simulink library "SEN"  (Simulink 10.2)
settings: Solver=VariableStepAuto  StartTime=0.0  StopTime=10.0  RelTol=1e-3
libraries: SEN_GYR x1, SEN_MTM x1, SEN_SPC x1, SEN_SUN x1
settings Model: Creator=dbell44  LastModifiedBy=dbell44

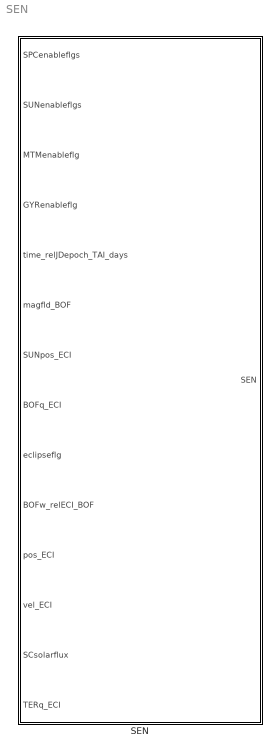
== system SEN ==
  SEN : Subsystem

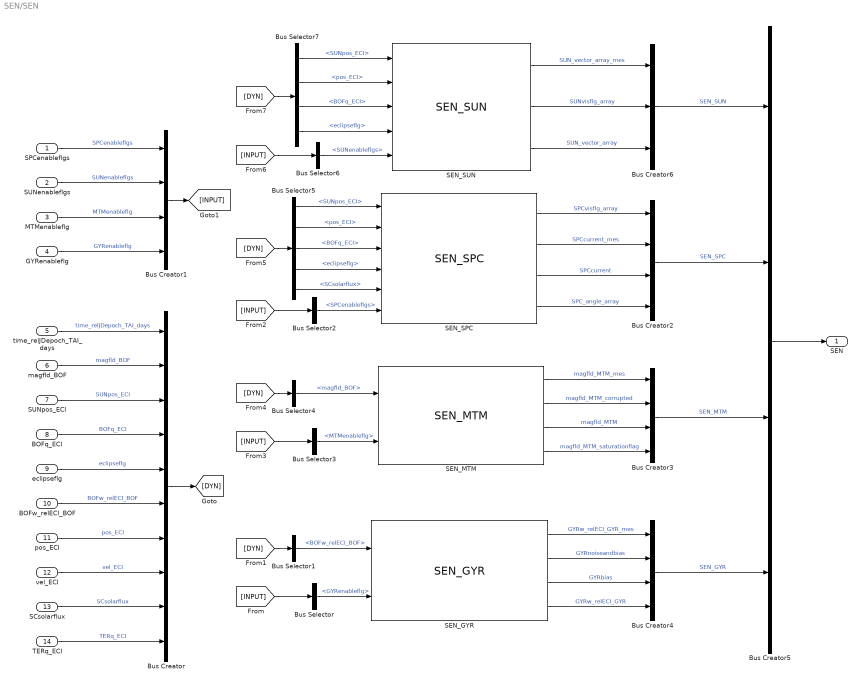
== system SEN/SEN ==
  SPCenableflgs : Inport
  SUNenableflgs : Inport  Port=2
  MTMenableflg : Inport  Port=3
  GYRenableflg : Inport  Port=4
  time_relJDepoch_TAI_days : Inport  Port=5
  magfld_BOF : Inport  Port=6
  SUNpos_ECI : Inport  Port=7
  BOFq_ECI : Inport  Port=8
  eclipseflg : Inport  Port=9
  BOFw_relECI_BOF : Inport  Port=10
  pos_ECI : Inport  Port=11
  vel_ECI : Inport  Port=12
  SCsolarflux : Inport  Port=13
  TERq_ECI : Inport  Port=14
  Bus Creator : BusCreator  Inputs=10
  Bus Creator{1..5} (5 alike) : BusCreator  Inputs=4
  Bus Creator6 : BusCreator  Inputs=3
  Bus Selector : BusSelector  OutputSignals=GYRenableflg
  Bus Selector1 : BusSelector  OutputSignals=BOFw_relECI_BOF
  Bus Selector2 : BusSelector  OutputSignals=SPCenableflgs
  Bus Selector3 : BusSelector  OutputSignals=MTMenableflg
  Bus Selector4 : BusSelector  OutputSignals=magfld_BOF
  Bus Selector5 : BusSelector  OutputSignals=SUNpos_ECI,pos_ECI,BOFq_ECI,eclipseflg,SCsolarflux
  Bus Selector6 : BusSelector  OutputSignals=SUNenableflgs
  Bus Selector7 : BusSelector  OutputSignals=SUNpos_ECI,pos_ECI,BOFq_ECI,eclipseflg
  SEN_GYR : SEN_GYR/SEN_GYR  SystemSampleTime=-1  VariantActivationTime=update diagram  Latency=0  AutoFrameSizeCalculation=off
  SEN_MTM : SEN_MTM/SEN_MTM  SystemSampleTime=-1  VariantActivationTime=update diagram  Latency=0  AutoFrameSizeCalculation=off
  SEN_SPC : SEN_SPC/SEN_SPC  SystemSampleTime=-1  VariantActivationTime=update diagram  Latency=0  AutoFrameSizeCalculation=off
  SEN_SUN : SEN_SUN/SEN_SUN  SystemSampleTime=-1  VariantActivationTime=update diagram  Latency=0  AutoFrameSizeCalculation=off
  SEN : Outport
  wires:
  time_relJDepoch_TAI_days/1 -> Bus Creator/1  "time_relJDepoch_TAI_days"
  magfld_BOF/1 -> Bus Creator/2  "magfld_BOF"
  SUNpos_ECI/1 -> Bus Creator/3  "SUNpos_ECI"
  BOFq_ECI/1 -> Bus Creator/4  "BOFq_ECI"
  eclipseflg/1 -> Bus Creator/5  "eclipseflg"
  BOFw_relECI_BOF/1 -> Bus Creator/6  "BOFw_relECI_BOF"
  pos_ECI/1 -> Bus Creator/7  "pos_ECI"
  vel_ECI/1 -> Bus Creator/8  "vel_ECI"
  SCsolarflux/1 -> Bus Creator/9  "SCsolarflux"
  TERq_ECI/1 -> Bus Creator/10  "TERq_ECI"
  Bus Creator/1 -> [DYN]
  SPCenableflgs/1 -> Bus Creator1/1  "SPCenableflgs"
  SUNenableflgs/1 -> Bus Creator1/2  "SUNenableflgs"
  MTMenableflg/1 -> Bus Creator1/3  "MTMenableflg"
  GYRenableflg/1 -> Bus Creator1/4  "GYRenableflg"
  Bus Creator1/1 -> [INPUT]
  [INPUT] -> Bus Selector/1
  Bus Selector/1 -> SEN_GYR/2  "<GYRenableflg>"
  [DYN] -> Bus Selector1/1
  Bus Selector1/1 -> SEN_GYR/1  "<BOFw_relECI_BOF>"
  SEN_GYR/1 -> Bus Creator4/1  "GYRw_relECI_GYR_mes"
  SEN_GYR/2 -> Bus Creator4/2  "GYRnoiseandbias"
  SEN_GYR/3 -> Bus Creator4/3  "GYRbias"
  SEN_GYR/4 -> Bus Creator4/4  "GYRw_relECI_GYR"
  Bus Selector4/1 -> SEN_MTM/1  "<magfld_BOF>"
  [INPUT] -> Bus Selector3/1
  Bus Selector3/1 -> SEN_MTM/2  "<MTMenableflg>"
  [DYN] -> Bus Selector4/1
  SEN_MTM/2 -> Bus Creator3/2  "magfld_MTM_corrupted"
  SEN_MTM/3 -> Bus Creator3/3  "magfld_MTM"
  SEN_MTM/4 -> Bus Creator3/4  "magfld_MTM_saturationflag"
  SEN_MTM/1 -> Bus Creator3/1  "magfld_MTM_mes"
  [INPUT] -> Bus Selector2/1
  Bus Selector2/1 -> SEN_SPC/6  "<SPCenableflgs>"
  [DYN] -> Bus Selector5/1
  Bus Selector5/1 -> SEN_SPC/1  "<SUNpos_ECI>"
  Bus Selector5/2 -> SEN_SPC/2  "<pos_ECI>"
  Bus Selector5/3 -> SEN_SPC/3  "<BOFq_ECI>"
  Bus Selector5/4 -> SEN_SPC/4  "<eclipseflg>"
  Bus Selector5/5 -> SEN_SPC/5  "<SCsolarflux>"
  SEN_SPC/1 -> Bus Creator2/1  "SPCvisflg_array"
  SEN_SPC/2 -> Bus Creator2/2  "SPCcurrent_mes"
  SEN_SPC/4 -> Bus Creator2/4  "SPC_angle_array"
  SEN_SPC/3 -> Bus Creator2/3  "SPCcurrent"
  Bus Selector7/1 -> SEN_SUN/1  "<SUNpos_ECI>"
  Bus Selector7/2 -> SEN_SUN/2  "<pos_ECI>"
  Bus Selector7/4 -> SEN_SUN/4  "<eclipseflg>"
  Bus Selector6/1 -> SEN_SUN/5  "<SUNenableflgs>"
  [INPUT] -> Bus Selector6/1
  [DYN] -> Bus Selector7/1
  Bus Selector7/3 -> SEN_SUN/3  "<BOFq_ECI>"
  SEN_SUN/2 -> Bus Creator6/2  "SUNvisflg_array"
  SEN_SUN/3 -> Bus Creator6/3  "SUN_vector_array"
  SEN_SUN/1 -> Bus Creator6/1  "SUN_vector_array_mes"
  Bus Creator5/1 -> SEN/1
  Bus Creator6/1 -> Bus Creator5/1  "SEN_SUN"
  Bus Creator2/1 -> Bus Creator5/2  "SEN_SPC"
  Bus Creator4/1 -> Bus Creator5/4  "SEN_GYR"
  Bus Creator3/1 -> Bus Creator5/3  "SEN_MTM"
